simulink model "beachball"  (R2022b)
settings: Solver=VariableStepAuto  StartTime=0.0  StopTime=10.0  RelTol=1e-3
libraries: VACLib x9
settings Model: Creator=KarlO  LastModifiedBy=KarlO

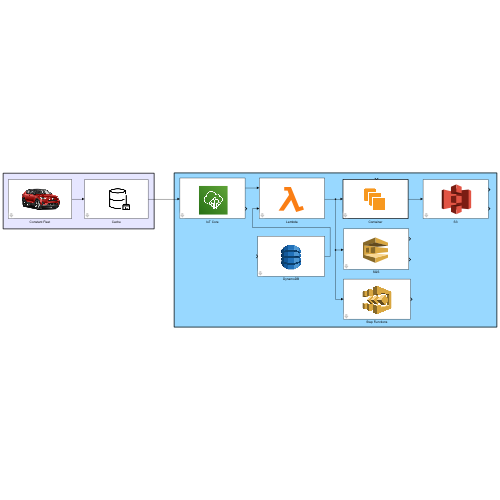
[thumbnail: Simulink's stored preview of the top-level diagram]
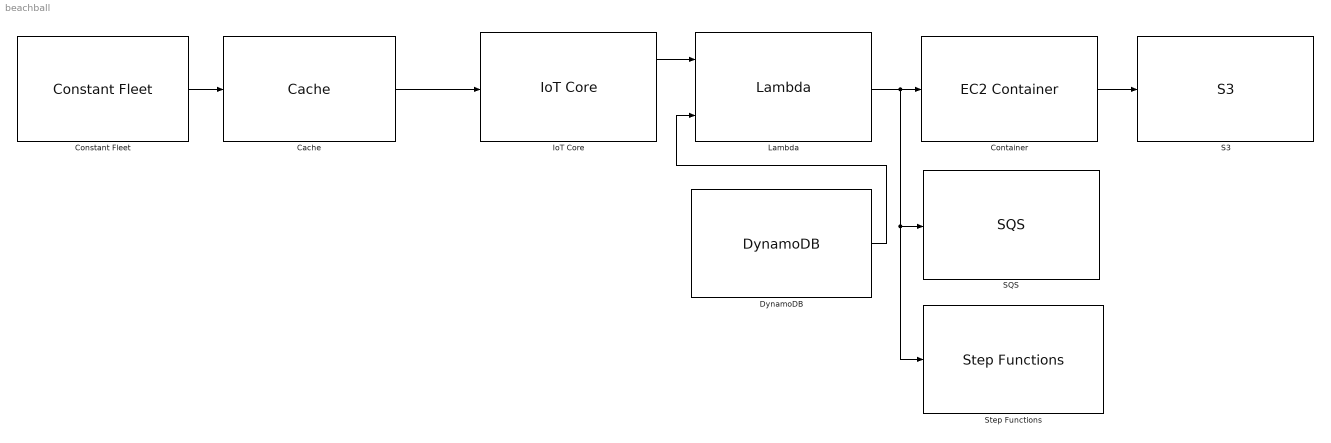
== system beachball ==
  Cache : VACLib/Vehicle Components/Cache  cache_size=0
      settings: SourceProductName=Volvo Architechture Components
  Constant Fleet : VACLib/Vehicle Components/Constant Fleet  time=10  frequency=1  fleet_size=0
      settings: SourceProductName=Volvo Architechture Components
  Container : VACLib/AWS Components/EC2 Container  no_cores=1  ram=8  no_instances=1
      settings: LibrarySourceBlock=|
      | simulink/User-Defined
      | Functions/MATLAB Function
  DynamoDB : VACLib/AWS Components/DynamoDB
      settings: SourceProductName=Volvo Architechture Components
  IoT Core : VACLib/AWS Components/IoT Core
      settings: SourceProductName=Volvo Architechture Components
  Lambda : VACLib/AWS Components/Lambda  parallel_instances=0  lambda_chunk_size=0
      settings: SourceProductName=Volvo Architechture Components
  S3 : VACLib/AWS Components/S3
      settings: SourceProductName=Volvo Architechture Components
  SQS : VACLib/AWS Components/SQS  queue_size=0  timeout=0
      settings: SourceProductName=Volvo Architechture Components
  Step Functions : VACLib/AWS Components/Step Functions
      settings: SourceProductName=Volvo Architechture Components
  wires:
  Constant Fleet/1 -> Cache/1
  Lambda/1 -> Step Functions/1, SQS/1, Container/1
  Cache/1 -> IoT Core/1
  IoT Core/1 -> Lambda/1
  DynamoDB/1 -> Lambda/2
  Container/1 -> S3/1
